simulink model "bouncingball"  (R2021a)
settings: Solver=ode1  StartTime=0.0  StopTime=25  FixedStep=0.1  RelTol=1e-3
settings Model: OrderedModelArguments=off  Creator=runnily  LastModifiedBy=runnily

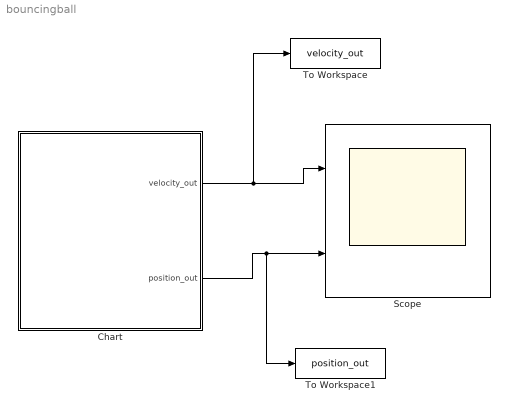
== system bouncingball ==
  Chart : Stateflow chart  TreatAsAtomicUnit=on
  Scope : Scope  NumInputPorts=2
  To Workspace : ToWorkspace  VariableName=velocity_out  SaveFormat=Structure With Time  SampleTime=0.1
  To Workspace1 : ToWorkspace  VariableName=position_out  SaveFormat=Structure With Time  SampleTime=0.1
  wires:
  Chart/1(velocity_out) -> To Workspace/1, Scope/1
  Chart/2(position_out) -> To Workspace1/1, Scope/2

== stateflow chart bouncingball/Chart ==
  settings: updateMethod=CONTINUOUS
  state Falling
    during:
    velocity_dot = -9.81;
    position_dot = velocity;
    position_out = position;
    velocity_out = velocity;
  (default) -> Falling : {position = 9.74;
      | velocity = 16;}
  Falling -> Falling : [position <= 0 && velocity <0]
      | { position = 0;
      |   velocity = -0.8*velocity;
      | }
  data: position local; velocity local; velocity_out output double; position_out output double
  data position settings: updateMethod=SF_CONTINUOUS_TIME_DATA
  data velocity settings: updateMethod=SF_CONTINUOUS_TIME_DATA
